simulink model "using_ros_matlab"  (R2021a)
settings: Solver=ode15s  StartTime=0.0  StopTime=60  RelTol=1e-3
libraries: robotlib x2, aerolibanimutils x1
settings Model: Creator=user  LastModifiedBy=user

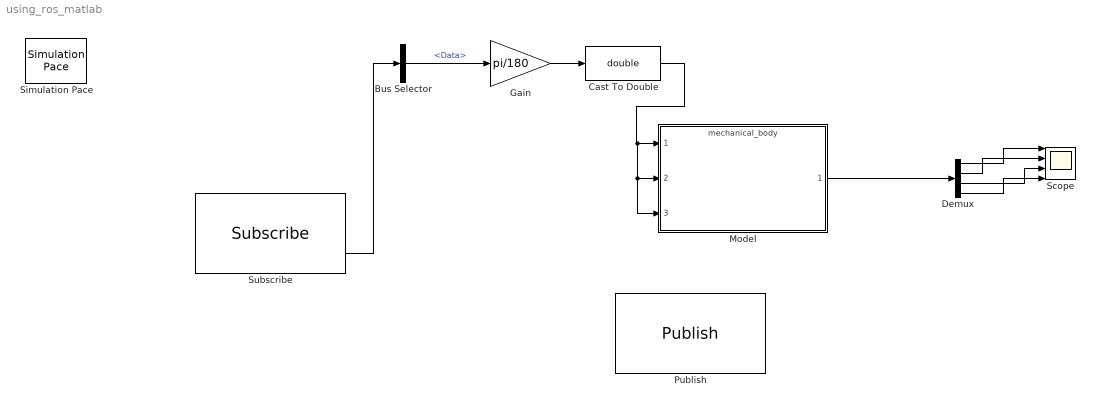
== system using_ros_matlab ==
  Bus Selector : BusSelector  OutputSignals=Data
  Cast To Double : DataTypeConversion  OutDataTypeStr=double
  Demux : Demux
  Gain : Gain  Gain=pi/180
  Model : ModelReference  ModelNameDialog=mechanical_body.slx  SimulationMode=Normal  ModelReferenceVersion=1.8
  Publish : robotlib/Publish  topicSource=Select from ROS network  topic=/my_topic  messageType=geometry_msgs/Point  legacyBusStruct=off  messageQueueLength=1
  Scope : Scope  NumInputPorts=4
  Simulation Pace : aerolibanimutils/Simulation Pace  SimulationPace=1  SleepMode=Auto  OutputPaceError=off  SampleTime=1/30
  Subscribe : robotlib/Subscribe  topicSource=Specify your own  topic=/joystick_topic  messageType=std_msgs/Int32  SampleTime=0.01  legacyBusStruct=off  messageQueueLength=1
  wires:
  Subscribe/2 -> Bus Selector/1
  Bus Selector/1 -> Gain/1  "<Data>"
  Gain/1 -> Cast To Double/1
  Cast To Double/1 -> Model/3, Model/2, Model/1
  Model/1 -> Demux/1
  Demux/1 -> Scope/1
  Demux/2 -> Scope/2
  Demux/3 -> Scope/3
  Demux/4 -> Scope/4
